simulink model "SLUGS2"  (R2015a)
settings: Solver=FixedStepDiscrete  StartTime=0.0  StopTime=10.0  FixedStep=T  RelTol=1e-3
PreLoadFcn:
  | %T = 0.0025;
  | MavlinkBus;
  | mcuInit;
  | % Baro Altitude Computation
  | % =========================
  | %basePressure = 98192.64;
  | %baseTemp = 288.215;
  | %lapseRate = -0.00198122;
  | %baseHeight = 0;
values from neighbouring files (symbols this model uses):
  apSampleTime = 0.01    [mcuInit.m]
  latlong_WP = 1    [mcuInit.m]
  mavlink_attitude_t = Simulink.Bus    [MavlinkBusMarcello.m]
  mavlink_gps_raw_int_t = Simulink.Bus    [MavlinkBus.m]    (also in MavlinkBusMarcello.m)
  mavlink_raw_imu_t = Simulink.Bus    [MavlinkBus.m]    (also in MavlinkBusMarcello.m)
  mavlink_scaled_pressure_t = Simulink.Bus    [MavlinkBus.m]    (also in MavlinkBusMarcello.m)
  mavlink_servo_output_raw_t = Simulink.Bus    [MavlinkBusMarcello.m]
  mavlink_slugs_navigation_t = Simulink.Bus    [MavlinkBusMarcello.m]
  mavlink_sys_status_t = Simulink.Bus    [MavlinkBus.m]    (also in MavlinkBusMarcello.m)
  SYS_ID_DEF = mpt.Parameter    [mcuInit.m]
  T = 0.01    [mcuInit.m]
  Xpoints = [0 0]    [mcuInit.m]
  Ypoints = [0 0]    [mcuInit.m]
  Zpoints = [0 0]    [mcuInit.m]
undefined symbols (not defined in the file or in its folder): A0, A14, A15, A2, A3, A4, A5, A6, accBiasRateLimit, B0, bankCommandLimit, barAdjust, baroCutoff, baroCutTemp, baseHeight, baseTemp, bdt, cubeAccelGain16405, cubeGyroGain16405, cubeMagGain16405, D0, D11, D7, D8, daLimit, data, daTrimMax, daTrimMin, deLimit, deTrimMax, deTrimMin, drLimit, drTrimMax, drTrimMin, dtLimit, dtTrimMax, dtTrimMin, F2, F3, G0, G13, G15, gaind, GS_location, gyroBiasRateLimit, imuOffset_xacc, imuOffset_xgyro, imuOffset_yacc, imuOffset_ygyro, imuOffset_zacc, imuOffset_zgyro, IPStar, ISA_g, Max, maxAcc, MaxDwnPthStar, maxDynPressure, maxEta, mdt, mlParamInterface ... (+34)
undefined symbols (not defined in the file): baroOffset, baroScale, barTGain1, barTGain2, barTMean1, barTMean2, bda, bde, bdr, bICda, bICde, bICdr, bICdt, derivativesConstant, lapseRate, lowRateSensorCutoff, mainSensorCutoff, mda, mde, mdr, mICda, mICde, mICdr, mICdt, pitotOffset, pitotScale, pitTGain1, pitTGain2, pitTMean1, pitTMean2, powerOffset, powerScale, pressureSensorCutoff, tempOffset, tempScale, vzCutoff, xCutoff, yCutoff
libraries: MCHP_Blockset x151, simulink x84, SLUGS_Library x31, aerolibconvert2 x6, aerolibutil x4, aerolibtransform2 x3, dspmtrx3 x2, aerolibobsolete x2
(part 19 of 24)

== system SLUGS2/Sensor_Data_Adapter/Sensor Suite/If no HIL then Read all the Sensors/if GPS is Ublox ==
  Enable : EnablePort
  Produce the GPS Main Data and update the AP State (lat lon hei cog sog) [gpsUblox.c]1 : MCHP_Blockset/User Functions/C Function Call  ParseFilesChkbx=on  ListFunctions1=Custom Function  Function1=void getGpsUbloxMainData(real32_T* y1);  AddHeaderDeclaration=on  Function1Type=when block is updated (default)  FctReturnBlockOut=off  Fct1BlockOut=y1[5]  DataCollected="s.chksm=reshape({ '638530-ספט-2016 08:52:24','251930-ספט-2016 08:52:57','1628430-ספט-2016 08:52:57','3862408-אוק-2016 23:39:15','360330-ספט-2016 08:52:57','7293730-ספט-2016 08:52:57','954930-ספט-2016 08:52:57','296108-אוק-2016 23:39:15','278130-ספט-2016 08:52:57','556030-ספט-2016 08:52:57','963230-ספט-2016 08:52:57','1122730-ספט-2016 08:52:57','372430-ספט-2016 08:52:57','998830-ספט-2016 08:52:57','522508-אוק-2016 23:39:15'},1,15);s.File1=reshape({ '  void  newCircBuffer(CBRef cB)','  void  freeCircBuffer(CBRef* cB)','  void  freeCircBuffer(CBRef* cB)',' unsigned int  getLength(CBRef cB)','  int  readHead(CBRef cB)','  int  readTail(CBRef cB)',' unsigned char  peak(CBRef cB)',' unsigned char  readFront(CBRef cB)',' unsigned char  writeBack(CBRef cB, unsigned char data)','  void  makeEmpty(CBRef cB)','  void  printCircBuf(CBRef cB)'},1,11);s.File2=reshape({ '  void  uartBufferInit(void)','  void  __attribute__((__interrupt__, no_auto_psv)) _U4RXInterrupt(void)','  void  getGPSRawData(unsigned char* gpsBuffer)',' unsigned char  isGPSNovatel(void)'},1,4);s.File3=reshape({ '  char  hex2char(char halfhex)','  float  degMinToDeg(unsigned char degrees, float minutes)',' unsigned char  gpsUbloxSeparate(unsigned char* outStream)','  void  gpsUbloxParse(void)','  void  getGpsUbloxMainData(float* data)','  char  gpSmbl(char symbl)',' unsigned char  myTokenizer(char* stringToTokenize, char token, char * returnToken)','  void  parseRMC(unsigned char* stream)','  void  parseGGA(unsigned char* stream)',' unsigned char  getChecksum(unsigned char* sentence, unsigned char size)','  void  gpsDebugMsg(unsigned char buf)'},1,11);s.File4=reshape({ '  void  uartMavlinkBufferInit(void)','  void __attribute__((__interrupt__,__auto_psv__)) _U1RXInterrupt(void)','  uint8_t  isFinite(float s)','  void  InitParameterInterface(void)','  void  protDecodeMavlink(void)','  uint16_t  MissionInterfaceResponse(uint8_t system_id, uint8_t component_id)','  uint16_t  ParameterInterfaceResponse(uint8_t system_id, uint8_t component_id)','  uint16_t  PackHeartBeat(uint8_t system_id, uint8_t component_id)','  uint16_t  PackTextMsg(uint8_t system_id, uint8_t component_id, unsigned char buf)','  uint16_t  PackRawIMU(uint8_t system_id, uint8_t component_id, mavlink_raw_imu_t mlRawIMUData ,uint32_t time_usec)','  uint16_t  PackRawAttitude(uint8_t system_id, uint8_t component_id, mavlink_attitude_t mlAttitudeData ,uint32_t time_usec)','  uint16_t  PackGpsRawInt(uint8_t system_id, uint8_t component_id, mavlink_gps_raw_int_t mlRawGpsDataInt ,uint32_t time_usec)','  uint16_t  PackScaledPressure(uint8_t system_id, uint8_t component_id, mavlink_scaled_pressure_t mlAirData ,uint32_t time_usec)','  uint16_t  PackSysStatus(uint8_t system_id, uint8_t component_id, mavlink_sys_status_t mlSysStatus)','  uint16_t  PackRawServo(uint8_t system_id, uint8_t component_id, mavlink_servo_output_raw_t mlPwmCommands ,uint32_t time_usec)','  uint16_t  HIL_PackRawServo(uint8_t system_id, uint8_t component_id, mavlink_servo_output_raw_t mlPwmCommands ,uint32_t time_usec)','  uint16_t  PackRawRC(uint8_t system_id, uint8_t component_id, mavlink_rc_channels_raw_t mlRC_Commands ,uint32_t time_usec)','  uint16_t  PackVFR_HUD(uint8_t system_id, uint8_t component_id, mavlink_vfr_hud_t mlVfr_hud ,uint32_t time_usec)','  char  sendQGCDebugMessage(const char * dbgMessage, char severity, unsigned char* bytesToAdd, char positionStart)','  void  TxN_Data_OverU1(uint16_t N)','  void  TxN_Data_OverU4(uint16_t N)'},1,21);s.File5=reshape({ '  float  myAtan2(float num, float denom)','  float  myPow(float x, float toTheN)','  float  mySqrt(float x)','  float  myAbs(float x)','  float  myAtan(float x)','  float  myAsin(float x)','  float  mySin(float x)','  float  myCos(float x)','  float  myTan(float x)','  float  myAcos(float x)','  float  myExp(float x)','  void  hugeDelay(void)','  void  smallDelay(void)','  void  tinyDelay(void)','  void  printToUart2(const char *fmt, ...)'},1,15);s.File6=reshape({ '  void  sendTelemetryMavlink(unsigned char* dataOut)','  void  uart2Init(void)','  void  gsRead(unsigned char* gsChunk)','  void  prepareTelemetryMavlink(unsigned char* dataOut)','  void  prepareTelemetryMavlink(unsigned char* dataOut)','  void  sendTelemetryMavlink(unsigned char* dataOut)','  void  copyBufferToDMA1(unsigned char size)','  void  send2GS(unsigned char* protData)','  uint8_t  clearWaypointsFrom(uint8_t startingWp)','  void  addMessageToSpiOut(mavlink_message_t* msg)'},1,10);s.File7={ '  void  populateParameterInterface(void)'};s.File8={ '  void  mavlinkInit(void)'};s.File9=reshape({ '  void  updatePWM(unsigned short * PWMData)','  void  updatePWMTrim(unsigned short PWMData, unsigned char channel)','  void  updateLoad(uint8_t mcuLoad)','  void  updateEuler(float* newEuler)','  void  updatePQR(float* newPQR)',' unsigned char  getHilOnOff(void)','  uint8_t  getLightsOnOff(void)','  uint8_t  getLightsDayNight(void)','  void  updateVISensor(uint16_t* data)','  void  updatePTZ(int16_t* ptz)'},1,10);s.File10=reshape({ '  void  updateRawADCData(int16_t* adcData)','  void  updateAirData(float* airData)','  void  updateLoadData(uint8_t load, uint16_t mvPower)','  void  updateAttitude(float * attitudeData)','  void  getGSLocation(float* altLatLon)','  void  updateTimeStamp(uint32_t timeSt)','  void  updatePosition(float * posData)','  void  updatePilotConsole(uint16_t * pilData)','  void  updateDiagnosticFl(float* diagFl)','  void  updateDiagnosticSh(int16_t* diagSh)','  void  updateBias(float * biasData)','  void  updateSensorData(float* sens)','  uint8_t  isFixValid(void)','  void  updateSensorDiag(float* diag)'},1,14);s.File11=reshape({ '  void  gpsInit(void)','  void  gpsParse(uint8_t* dataStream)','  void  updateStatus(uint8_t* completeMessage)','  void  updatePositionData(uint8_t* completeMessage)','  void  updateVelocityData(uint8_t* completeMessage)','  void  updateTimeData(uint8_t* completeMessage)','  void  getGpsMainData(float* data)','  uint32_t  CRC32Value(int32_t i)','  uint32_t  CalculateBlockCRC32(uint32_t ulCount, uint8_t *ucBuffer)','  uint16_t  charsToUint16(uint8_t* data)','  uint32_t  charsToUint32(uint8_t* data)','  float  charsToFloat(uint8_t* data)','  double  charsToDouble(uint8_t* data)'},1,13);s.File12=reshape({ '  void  getMidLevelCommands(float* commands)',' unsigned char  isApManual(uint16_t failsafe)','  float  getParamIdx(unsigned char idx)','  void  getRangeOfParams(uint8_t startIdx, uint8_t endIdx, float* parameters)','  float  getDynamic(void)','  void  getAttitude(float* attitude)','  void  getXYZ(float* xyz)','  void  getVned(float* xyz)','  uint8_t  getMaxWp(void)',' unsigned char  isWpFly(void)',' unsigned char  isPassthrough(void)','  void  setDiagnosticFloat(float * flValues)','  void  setDiagnosticShort(int16_t* shValues)','  void  getWP(unsigned char idx, float* WPpos)','  void  setLogFloat1(float * flValues)','  void  setLogFloat2(float * flValues)',' unsigned char  getApControlType(void)',' unsigned char  getPassValues(uint8_t* pasVals)','  void  setCurrentCommands(float airSpeed)','  void  getCurrentGPSPos(float* latLonAlt)','  void  setNavLong(float* values)','  void  setNavLat(float* values)','  void  setNavNav(float* values)','  void  getAccels(float * accels)','  void  getAccBias(float * bias)','  void  getRTB(uint8_t* rtb)','  void  getMobileLocation(float* loc)','  uint8_t  getNavMode(void)','  void  getISRLocation(float* loc)','  uint8_t  getISRCameraOption1(void)',' unsigned short  meanFilter5(unsigned short * values)','  uint8_t  justEnabled(uint8_t enableValue, uint8_t index)',' unsigned char  quickSort(unsigned short *arr, char elements)'},1,33);s.File13=reshape({ '  void  hilRead(unsigned char* hilChunk)','  void  hil_getRawRead(short * rawData)','  void  hil_getVned(float* vned)','  void  hil_getEuler(float* euler)','  void  hil_getRates(float* pqr)','  void  hil_getXYZ(float* xyz)',' unsigned int  hil_getTs(void)','  void  protDecodeHil(uint8_t* dataIn)'},1,8);s.File14=reshape({ '  void  cubeInit(void)','  void  getCubeData(short * cubeData)','  void  updateCubeData(void)','  int16_t  averageData(int16_t* theData, uint8_t count)',' unsigned short  write2Cube(unsigned short data2Send)','  short  convert14BitToShort(short wordData)','  short  convert12BitToShort(short wordData)',' unsigned char  isCube16405(void)'},1,8);s.File15=reshape({ '  void  uartMavlinkBufferInit(void)','  uint16_t  PackHeartBeat(uint8_t system_id, uint8_t component_id)','  uint16_t  PackRawServo(uint8_t system_id, uint8_t component_id, mavlink_servo_output_raw_t mlPwmCommands ,uint32_t time_usec)','  uint16_t  HIL_PackRawServo(uint8_t system_id, uint8_t component_id, mavlink_servo_output_raw_t mlPwmCommands ,uint32_t time_usec)','  uint16_t  PackRawRC(uint8_t system_id, uint8_t component_id, mavlink_rc_channels_raw_t mlRC_Commands, uint32_t time_usec)','  uint16_t  PackVFR_HUD(uint8_t system_id, uint8_t component_id, mavlink_vfr_hud_t mlVfr_hud, uint32_t time_usec)','  uint16_t  PackRawIMU(uint8_t system_id, uint8_t component_id, mavlink_raw_imu_t mlRawIMUData ,uint32_t time_usec)','  uint16_t  PackRawAttitude(uint8_t system_id, uint8_t component_id, mavlink_attitude_t mlAttitudeData ,uint32_t time_usec)','  char  sendQGCDebugMessage(const char * dbgMessage, char severity, unsigned char* bytesToAdd, char positionStart)','  uint16_t  PackGpsRawInt(uint8_t system_id, uint8_t component_id, mavlink_gps_raw_int_t mlRawGpsDataInt, uint32_t time_usec)','  uint16_t  PackScaledPressure(uint8_t system_id, uint8_t component_id, mavlink_scaled_pressure_t mlAirData, uint32_t time_usec)','  uint16_t  PackSysStatus(uint8_t system_id, uint8_t component_id, mavlink_sys_status_t mlSysStatus)'},1,12);"  ORDERING=None  SampleTime=.01  MCHP_MASTERLINK=|  PinDigitalInput=[]  PinDigitalOutput=[]  PinAnalogInput=[]
      | SLUGS2/Microchip Master
      | AUAV V3 Board
      | Busy Flag on D2 (RA6)
  GPS Main : Outport
  wires:
  Produce the GPS Main Data and update the AP State (lat lon hei cog sog) [gpsUblox.c]1/1 -> GPS Main/1

== system SLUGS2/Sensor_Data_Adapter/Sensor Suite/Low Pass Filtering,Temperature Compensation and Calibration/Baro Altimeter ==
  Static (Pa) : Inport
  Compute Barometric Height : Subsystem  mask{baseTemp=baseTemp, LapseRate=lapseRate}
      mask prompts: baseTemp "Base Station Temperature (K)"; LapseRate "Lapse Rate (C/ft)"
      mask help:
      | Produces Altitude in meters from Barometric Pressure in Pascals. Altitude is valid from MSL to 6000 ft.
      |
      | The method implemented here was developed by Ren Curry
  Enabled Subsystem : Subsystem  TreatAsAtomicUnit=on
  Enables/Disables the Computation of initial Baro Bias : MATLAB Function  TreatAsAtomicUnit=on
  GS Height : Subsystem
  Initial Baro Bias : Subsystem  TreatAsAtomicUnit=on
  Logical Operator : Logic  Operator=NOT  AllPortsSameDT=off  OutDataTypeStr=boolean
  Sum1 : Sum  Inputs=++|  OutDataTypeStr=single
  Zero Out Height : Subsystem  TreatAsAtomicUnit=on
  Altitude : Outport
  wires:
  Compute Barometric Height/1("Altitude, m") -> Zero Out Height/2(Computed Height), Sum1/2
  Static (Pa)/1 -> Initial Baro Bias/1(Baro (Pa)), Compute Barometric Height/3(Baro (Pa))
  Enables/Disables the Computation of initial Baro Bias/1(tOut) -> Initial Baro Bias/Enable, Zero Out Height/Enable, Logical Operator/1
  GS Height/1(GS Height) -> Compute Barometric Height/1(Base Height (m)), Zero Out Height/1(Base Height)
  Initial Baro Bias/1(Baro (Gnd)) -> Compute Barometric Height/2(Base Pressure (Pa))
  Zero Out Height/1(Height Offset) -> Sum1/1
  Logical Operator/1 -> Enabled Subsystem/Enable
  Sum1/1 -> Enabled Subsystem/1(In1)
  Enabled Subsystem/1(Out1) -> Altitude/1

== system SLUGS2/Sensor_Data_Adapter/Sensor Suite/Low Pass Filtering,Temperature Compensation and Calibration/Barometer Unit Conversion ==
  Raw : Inport
  Bias : Constant  Value=bias  OutDataTypeStr=single
  Divide : Product  OutDataTypeStr=single
  Gains : Constant  Value=gains  OutDataTypeStr=single
  Sum : Sum  Inputs=|++  OutDataTypeStr=single
  Comp : Outport
  wires:
  Bias/1 -> Sum/2
  Raw/1 -> Divide/2
  Gains/1 -> Divide/1
  Divide/1 -> Sum/1
  Sum/1 -> Comp/1

== system SLUGS2/Sensor_Data_Adapter/Sensor Suite/Low Pass Filtering,Temperature Compensation and Calibration/Pitot Unit Conversion ==
  Raw : Inport
  Bias : Constant  Value=bias  OutDataTypeStr=single
  Divide : Product  OutDataTypeStr=single
  Gains : Constant  Value=gains  OutDataTypeStr=single
  Sum : Sum  Inputs=|++  OutDataTypeStr=single
  Comp : Outport
  wires:
  Bias/1 -> Sum/2
  Raw/1 -> Divide/2
  Gains/1 -> Divide/1
  Divide/1 -> Sum/1
  Sum/1 -> Comp/1

== system SLUGS2/Sensor_Data_Adapter/Sensor Suite/Low Pass Filtering,Temperature Compensation and Calibration/Power Unit Conversion ==
  Raw : Inport
  Bias : Constant  Value=bias  OutDataTypeStr=single
  Divide : Product  OutDataTypeStr=single
  Gains : Constant  Value=gains  OutDataTypeStr=single
  Sum : Sum  Inputs=|++  OutDataTypeStr=single
  Comp : Outport
  wires:
  Bias/1 -> Sum/2
  Raw/1 -> Divide/2
  Gains/1 -> Divide/1
  Divide/1 -> Sum/1
  Sum/1 -> Comp/1

== system SLUGS2/Sensor_Data_Adapter/Sensor Suite/Low Pass Filtering,Temperature Compensation and Calibration/Temp Compensate Accel X1 ==
  Temp : Inport
  Dynamic : Inport  Port=2
  Compare To Constant : simulink/Logic and Bit Operations/Compare To Constant  relop=<  const=pitCutTemp  OutDataTypeStr=uint8  ZeroCross=off
  Display : Display
  Display2 : Display
  Hi Temp Compensation2 : Subsystem  mask{alpha=pitTGain2, tempMean=pitTMean2}
      mask prompts: alpha "Tempearature Coeficient (K_t)"; tempMean "Calibration Temperature Mean (T_avg)"
      mask help:
      | This block implements a temperature compensation. It implmements the following equation:
      |
      | M_tc = M_raw - K_t(T - T_avg)
  Lo Temp Compensation : Subsystem  mask{alpha=pitTGain1, tempMean=pitTMean1}
      mask prompts: alpha "Tempearature Coeficient (K_t)"; tempMean "Calibration Temperature Mean (T_avg)"
      mask help:
      | This block implements a temperature compensation. It implmements the following equation:
      |
      | M_tc = M_raw - K_t(T - T_avg)
  Logical Operator : Logic  Operator=NOT  AllPortsSameDT=off  OutDataTypeStr=boolean
  Merge : Merge
  Baro_c : Outport
  wires:
  Hi Temp Compensation2/1(Comp) -> Merge/1
  Logical Operator/1 -> Hi Temp Compensation2/Enable, Display2/1
  Merge/1 -> Baro_c/1, Display/1
  Dynamic/1 -> Lo Temp Compensation/1(Raw), Hi Temp Compensation2/1(Raw)
  Temp/1 -> Compare To Constant/1, Lo Temp Compensation/2(Temp Raw), Hi Temp Compensation2/2(Temp Raw)
  Compare To Constant/1 -> Lo Temp Compensation/Enable, Logical Operator/1
  Lo Temp Compensation/1(Comp) -> Merge/2

== system SLUGS2/Sensor_Data_Adapter/Sensor Suite/Low Pass Filtering,Temperature Compensation and Calibration/Temp Compensate Baro ==
  Temp : Inport
  Baro : Inport  Port=2
  Compare To Constant : simulink/Logic and Bit Operations/Compare To Constant  relop=<  const=baroCutTemp  OutDataTypeStr=uint8  ZeroCross=off
  Hi Temp Compensation : Subsystem  mask{alpha=barTGain2, tempMean=barTMean2}
      mask prompts: alpha "Tempearature Coeficient (K_t)"; tempMean "Calibration Temperature Mean (T_avg)"
      mask help:
      | This block implements a temperature compensation. It implmements the following equation:
      |
      | M_tc = M_raw - K_t(T - T_avg)
  Lo Temp Compensation : Subsystem  mask{alpha=barTGain1, tempMean=barTMean1}
      mask prompts: alpha "Tempearature Coeficient (K_t)"; tempMean "Calibration Temperature Mean (T_avg)"
      mask help:
      | This block implements a temperature compensation. It implmements the following equation:
      |
      | M_tc = M_raw - K_t(T - T_avg)
  Logical Operator : Logic  Operator=NOT  AllPortsSameDT=off  OutDataTypeStr=boolean
  Merge : Merge
  Baro_c : Outport
  wires:
  Compare To Constant/1 -> Logical Operator/1, Lo Temp Compensation/Enable
  Temp/1 -> Compare To Constant/1, Hi Temp Compensation/2(Temp Raw), Lo Temp Compensation/2(Temp Raw)
  Baro/1 -> Hi Temp Compensation/1(Raw), Lo Temp Compensation/1(Raw)
  Lo Temp Compensation/1(Comp) -> Merge/2
  Merge/1 -> Baro_c/1
  Logical Operator/1 -> Hi Temp Compensation/Enable
  Hi Temp Compensation/1(Comp) -> Merge/1

== system SLUGS2/Sensor_Data_Adapter/Sensor Suite/Low Pass Filtering,Temperature Compensation and Calibration/Thermistor Unit Conversion ==
  Raw : Inport
  Bias : Constant  Value=bias  OutDataTypeStr=single
  Divide : Product  OutDataTypeStr=single
  Gains : Constant  Value=gains  OutDataTypeStr=single
  Sum : Sum  Inputs=|++  OutDataTypeStr=single
  Comp : Outport
  wires:
  Sum/1 -> Comp/1
  Divide/1 -> Sum/1
  Gains/1 -> Divide/1
  Raw/1 -> Divide/2
  Bias/1 -> Sum/2

== system SLUGS2/Sensor_Data_Adapter/Sensor Suite/Low Pass Filtering,Temperature Compensation and Calibration/Tustin Lowpass, Auto Initial Condition1 ==
  In1 : Inport
  Constant : Constant  Value=T
  Constant1 : Constant  Value=f
  Embedded MATLAB Function : MATLAB Function  TreatAsAtomicUnit=on
  Out1 : Outport
  wires:
  Constant/1 -> Embedded MATLAB Function/2(T)
  Constant1/1 -> Embedded MATLAB Function/3(f)
  Embedded MATLAB Function/1(y) -> Out1/1
  In1/1 -> Embedded MATLAB Function/1(u)

== system SLUGS2/Sensor_Data_Adapter/Sensor Suite/Low Pass Filtering,Temperature Compensation and Calibration/Tustin Lowpass, Auto Initial Condition2 ==
  In1 : Inport
  Constant : Constant  Value=T
  Constant1 : Constant  Value=f
  Embedded MATLAB Function : MATLAB Function  TreatAsAtomicUnit=on
  Out1 : Outport
  wires:
  In1/1 -> Embedded MATLAB Function/1(u)
  Embedded MATLAB Function/1(y) -> Out1/1
  Constant1/1 -> Embedded MATLAB Function/3(f)
  Constant/1 -> Embedded MATLAB Function/2(T)

== system SLUGS2/Sensor_Data_Adapter/Sensor Suite/Low Pass Filtering,Temperature Compensation and Calibration/Tustin Lowpass, Auto Initial Condition3 ==
  In1 : Inport
  Constant : Constant  Value=T
  Constant1 : Constant  Value=f
  Embedded MATLAB Function : MATLAB Function  TreatAsAtomicUnit=on
  Out1 : Outport
  wires:
  Constant/1 -> Embedded MATLAB Function/2(T)
  Constant1/1 -> Embedded MATLAB Function/3(f)
  Embedded MATLAB Function/1(y) -> Out1/1
  In1/1 -> Embedded MATLAB Function/1(u)

== system SLUGS2/Sensor_Data_Adapter/Sensor Suite/Low Pass Filtering,Temperature Compensation and Calibration/Tustin Lowpass, Auto Initial Condition4 ==
  In1 : Inport
  Constant : Constant  Value=T
  Constant1 : Constant  Value=f
  Embedded MATLAB Function : MATLAB Function  TreatAsAtomicUnit=on
  Out1 : Outport
  wires:
  In1/1 -> Embedded MATLAB Function/1(u)
  Embedded MATLAB Function/1(y) -> Out1/1
  Constant1/1 -> Embedded MATLAB Function/3(f)
  Constant/1 -> Embedded MATLAB Function/2(T)

== system SLUGS2/Update PWM Commands and Send Telemetry [updated 4.27.16]/Generate PWM Signals Based on the Control Type/If  Control Type Is Selective Passthrough/Convert to PWM ==
  " Angle(rad)" : Inport
  Add : Sum
  Constant1 : Constant  Value=slopem
  Constant2 : Constant  Value=interceptb
  Data Type Conversion : DataTypeConversion  OutDataTypeStr=uint16
  Divide : Product
  PWM : Outport
  wires:
  Data Type Conversion/1 -> PWM/1
  " Angle(rad)"/1 -> Divide/1
  Constant2/1 -> Add/2
  Divide/1 -> Add/1
  Add/1 -> Data Type Conversion/1
  Constant1/1 -> Divide/2

== system SLUGS2/Update PWM Commands and Send Telemetry [updated 4.27.16]/Generate PWM Signals Based on the Control Type/If  Control Type Is Selective Passthrough/Convert to PWM1 ==
  " Angle(rad)" : Inport
  Add : Sum
  Constant1 : Constant  Value=slopem
  Constant2 : Constant  Value=interceptb
  Data Type Conversion : DataTypeConversion  OutDataTypeStr=uint16
  Divide : Product
  PWM : Outport
  wires:
  Constant1/1 -> Divide/2
  Add/1 -> Data Type Conversion/1
  Divide/1 -> Add/1
  Constant2/1 -> Add/2
  " Angle(rad)"/1 -> Divide/1
  Data Type Conversion/1 -> PWM/1

== system SLUGS2/Update PWM Commands and Send Telemetry [updated 4.27.16]/Generate PWM Signals Based on the Control Type/If  Control Type Is Selective Passthrough/Convert to PWM2 ==
  " Angle(rad)" : Inport
  Add : Sum
  Constant1 : Constant  Value=slopem
  Constant2 : Constant  Value=interceptb
  Data Type Conversion : DataTypeConversion  OutDataTypeStr=uint16
  Divide : Product
  PWM : Outport
  wires:
  Data Type Conversion/1 -> PWM/1
  " Angle(rad)"/1 -> Divide/1
  Constant2/1 -> Add/2
  Divide/1 -> Add/1
  Add/1 -> Data Type Conversion/1
  Constant1/1 -> Divide/2

== system SLUGS2/Update PWM Commands and Send Telemetry [updated 4.27.16]/Generate PWM Signals Based on the Control Type/If  Control Type Is Selective Passthrough/Convert to PWM3 ==
  " Angle(rad)" : Inport
  Add : Sum
  Constant1 : Constant  Value=slopem
  Constant2 : Constant  Value=interceptb
  Data Type Conversion : DataTypeConversion  OutDataTypeStr=uint16
  Divide : Product
  PWM : Outport
  wires:
  Constant1/1 -> Divide/2
  Add/1 -> Data Type Conversion/1
  Divide/1 -> Add/1
  Constant2/1 -> Add/2
  " Angle(rad)"/1 -> Divide/1
  Data Type Conversion/1 -> PWM/1

== system SLUGS2/Update PWM Commands and Send Telemetry [updated 4.27.16]/Generate PWM Signals Based on the Control Type/If  Control Type Is Wp, ISR, LP or  Mid Lvl Cmds/Convert to PWM ==
  " Angle(rad)" : Inport
  Add : Sum
  Constant1 : Constant  Value=slopem
  Constant2 : Constant  Value=interceptb
  Data Type Conversion : DataTypeConversion  OutDataTypeStr=uint16
  Divide : Product
  PWM : Outport
  wires:
  Data Type Conversion/1 -> PWM/1
  " Angle(rad)"/1 -> Divide/1
  Constant2/1 -> Add/2
  Divide/1 -> Add/1
  Add/1 -> Data Type Conversion/1
  Constant1/1 -> Divide/2

== system SLUGS2/Update PWM Commands and Send Telemetry [updated 4.27.16]/Generate PWM Signals Based on the Control Type/If  Control Type Is Wp, ISR, LP or  Mid Lvl Cmds/Convert to PWM1 ==
  " Angle(rad)" : Inport
  Add : Sum
  Constant1 : Constant  Value=slopem
  Constant2 : Constant  Value=interceptb
  Data Type Conversion : DataTypeConversion  OutDataTypeStr=uint16
  Divide : Product
  PWM : Outport
  wires:
  Constant1/1 -> Divide/2
  Add/1 -> Data Type Conversion/1
  Divide/1 -> Add/1
  Constant2/1 -> Add/2
  " Angle(rad)"/1 -> Divide/1
  Data Type Conversion/1 -> PWM/1

== system SLUGS2/Update PWM Commands and Send Telemetry [updated 4.27.16]/Generate PWM Signals Based on the Control Type/If  Control Type Is Wp, ISR, LP or  Mid Lvl Cmds/Convert to PWM2 ==
  " Angle(rad)" : Inport
  Add : Sum
  Constant1 : Constant  Value=slopem
  Constant2 : Constant  Value=interceptb
  Data Type Conversion : DataTypeConversion  OutDataTypeStr=uint16
  Divide : Product
  PWM : Outport
  wires:
  Data Type Conversion/1 -> PWM/1
  " Angle(rad)"/1 -> Divide/1
  Constant2/1 -> Add/2
  Divide/1 -> Add/1
  Add/1 -> Data Type Conversion/1
  Constant1/1 -> Divide/2

== system SLUGS2/Update PWM Commands and Send Telemetry [updated 4.27.16]/Generate PWM Signals Based on the Control Type/If  Control Type Is Wp, ISR, LP or  Mid Lvl Cmds/Convert to PWM3 ==
  " Angle(rad)" : Inport
  Add : Sum
  Constant1 : Constant  Value=slopem
  Constant2 : Constant  Value=interceptb
  Data Type Conversion : DataTypeConversion  OutDataTypeStr=uint16
  Divide : Product
  PWM : Outport
  wires:
  Constant1/1 -> Divide/2
  Add/1 -> Data Type Conversion/1
  Divide/1 -> Add/1
  Constant2/1 -> Add/2
  " Angle(rad)"/1 -> Divide/1
  Data Type Conversion/1 -> PWM/1

== system SLUGS2/Update PWM Commands and Send Telemetry [updated 4.27.16]/Generate PWM Signals Based on the Control Type/If  Control Type Is Wp, ISR, LP or  Mid Lvl Cmds and we want to add Selective Passthrough1/Average ==
  In1 : Inport
  In2 : Inport  Port=2
  Add : Sum
  Gain4 : Gain  Gain=1/2
  Out1 : Outport
  wires:
  In1/1 -> Add/1
  Gain4/1 -> Out1/1
  Add/1 -> Gain4/1
  In2/1 -> Add/2

== system SLUGS2/Update PWM Commands and Send Telemetry [updated 4.27.16]/Generate PWM Signals Based on the Control Type/If  Control Type Is Wp, ISR, LP or  Mid Lvl Cmds and we want to add Selective Passthrough1/Average1 ==
  In1 : Inport
  In2 : Inport  Port=2
  Add : Sum
  Gain4 : Gain  Gain=1/2
  Out1 : Outport
  wires:
  In1/1 -> Add/1
  Gain4/1 -> Out1/1
  Add/1 -> Gain4/1
  In2/1 -> Add/2

== system SLUGS2/Update PWM Commands and Send Telemetry [updated 4.27.16]/Generate PWM Signals Based on the Control Type/If  Control Type Is Wp, ISR, LP or  Mid Lvl Cmds and we want to add Selective Passthrough1/Average2 ==
  In1 : Inport
  In2 : Inport  Port=2
  Add : Sum
  Gain4 : Gain  Gain=1/2
  Out1 : Outport
  wires:
  In1/1 -> Add/1
  Gain4/1 -> Out1/1
  Add/1 -> Gain4/1
  In2/1 -> Add/2

== system SLUGS2/Update PWM Commands and Send Telemetry [updated 4.27.16]/Generate PWM Signals Based on the Control Type/If  Control Type Is Wp, ISR, LP or  Mid Lvl Cmds and we want to add Selective Passthrough1/Average3 ==
  In1 : Inport
  In2 : Inport  Port=2
  Add : Sum
  Gain4 : Gain  Gain=1/2
  Out1 : Outport
  wires:
  In1/1 -> Add/1
  Gain4/1 -> Out1/1
  Add/1 -> Gain4/1
  In2/1 -> Add/2

== system SLUGS2/Update PWM Commands and Send Telemetry [updated 4.27.16]/Generate PWM Signals Based on the Control Type/If  Control Type Is Wp, ISR, LP or  Mid Lvl Cmds and we want to add Selective Passthrough1/Convert to PWM ==
  " Angle(rad)" : Inport
  Add : Sum
  Constant1 : Constant  Value=slopem
  Constant2 : Constant  Value=interceptb
  Data Type Conversion : DataTypeConversion  OutDataTypeStr=uint16
  Divide : Product
  PWM : Outport
  wires:
  Data Type Conversion/1 -> PWM/1
  " Angle(rad)"/1 -> Divide/1
  Constant2/1 -> Add/2
  Divide/1 -> Add/1
  Add/1 -> Data Type Conversion/1
  Constant1/1 -> Divide/2

== system SLUGS2/Update PWM Commands and Send Telemetry [updated 4.27.16]/Generate PWM Signals Based on the Control Type/If  Control Type Is Wp, ISR, LP or  Mid Lvl Cmds and we want to add Selective Passthrough1/Convert to PWM1 ==
  " Angle(rad)" : Inport
  Add : Sum
  Constant1 : Constant  Value=slopem
  Constant2 : Constant  Value=interceptb
  Data Type Conversion : DataTypeConversion  OutDataTypeStr=uint16
  Divide : Product
  PWM : Outport
  wires:
  Constant1/1 -> Divide/2
  Add/1 -> Data Type Conversion/1
  Divide/1 -> Add/1
  Constant2/1 -> Add/2
  " Angle(rad)"/1 -> Divide/1
  Data Type Conversion/1 -> PWM/1

== system SLUGS2/Update PWM Commands and Send Telemetry [updated 4.27.16]/Generate PWM Signals Based on the Control Type/If  Control Type Is Wp, ISR, LP or  Mid Lvl Cmds and we want to add Selective Passthrough1/Convert to PWM2 ==
  " Angle(rad)" : Inport
  Add : Sum
  Constant1 : Constant  Value=slopem
  Constant2 : Constant  Value=interceptb
  Data Type Conversion : DataTypeConversion  OutDataTypeStr=uint16
  Divide : Product
  PWM : Outport
  wires:
  Data Type Conversion/1 -> PWM/1
  " Angle(rad)"/1 -> Divide/1
  Constant2/1 -> Add/2
  Divide/1 -> Add/1
  Add/1 -> Data Type Conversion/1
  Constant1/1 -> Divide/2

== system SLUGS2/Update PWM Commands and Send Telemetry [updated 4.27.16]/Generate PWM Signals Based on the Control Type/If  Control Type Is Wp, ISR, LP or  Mid Lvl Cmds and we want to add Selective Passthrough1/Convert to PWM3 ==
  " Angle(rad)" : Inport
  Add : Sum
  Constant1 : Constant  Value=slopem
  Constant2 : Constant  Value=interceptb
  Data Type Conversion : DataTypeConversion  OutDataTypeStr=uint16
  Divide : Product
  PWM : Outport
  wires:
  Constant1/1 -> Divide/2
  Add/1 -> Data Type Conversion/1
  Divide/1 -> Add/1
  Constant2/1 -> Add/2
  " Angle(rad)"/1 -> Divide/1
  Data Type Conversion/1 -> PWM/1

== system SLUGS2/Inner Loop// Navigation/L1 Output Feedback Controller With Projection Operator/Control Law/Compute Coef/dsPIC_exp ==
  u : Inport
  Environment Controller : simulink/Signal Routing/Environment Controller
  Math Function : Math  SaturateOnIntegerOverflow=on
  myExp() apUtils.c [updated 5.1.16] : MCHP_Blockset/User Functions/C Function Call  ParseFilesChkbx=off  ListFunctions1=Custom Function  Function1=float myExp(float x)  AddHeaderDeclaration=on  Function1Type=when block is updated (default)  Fct1BlockIn=x  FctReturnBlockOut=on  DataCollected=0  ORDERING=None  SampleTime=-1  MCHP_MASTERLINK=|  PinDigitalInput=[]  PinDigitalOutput=[]  PinAnalogInput=[]
      | SLUGS2/Microchip Master
      | AUAV V3 Board
      | Busy Flag on D2 (RA6)
  exp(u) : Outport
  wires:
  Math Function/1 -> Environment Controller/1
  u/1 -> Math Function/1, myExp() apUtils.c [updated 5.1.16]/1
  Environment Controller/1 -> exp(u)/1
  myExp() apUtils.c [updated 5.1.16]/1 -> Environment Controller/2

== system SLUGS2/Inner Loop// Navigation/L1 Output Feedback Controller With Projection Operator/State Predictor/Compute Coef/dsPIC_exp ==
  u : Inport
  Environment Controller : simulink/Signal Routing/Environment Controller
  Math Function : Math  SaturateOnIntegerOverflow=on
  myExp() apUtils.c [updated 5.1.16] : MCHP_Blockset/User Functions/C Function Call  ParseFilesChkbx=off  ListFunctions1=Custom Function  Function1=float myExp(float x)  AddHeaderDeclaration=on  Function1Type=when block is updated (default)  Fct1BlockIn=x  FctReturnBlockOut=on  DataCollected=0  ORDERING=None  SampleTime=-1  MCHP_MASTERLINK=|  PinDigitalInput=[]  PinDigitalOutput=[]  PinAnalogInput=[]
      | SLUGS2/Microchip Master
      | AUAV V3 Board
      | Busy Flag on D2 (RA6)
  exp(u) : Outport
  wires:
  Math Function/1 -> Environment Controller/1
  u/1 -> Math Function/1, myExp() apUtils.c [updated 5.1.16]/1
  Environment Controller/1 -> exp(u)/1
  myExp() apUtils.c [updated 5.1.16]/1 -> Environment Controller/2

== system SLUGS2/Inner Loop// Navigation/Lateral Channel Encaps [updated 4.28.16]/Lateral Channel/Roll Control [PID]/Trapezoidal Integrator ==
  x : Inport
  Reset : Inport  Port=2
  Constant : Constant  Value=1/3  OutDataTypeStr=single
  Constant1 : Constant  Value=4/3  OutDataTypeStr=single
  Constant2 : Constant  Value=T/2  OutDataTypeStr=single
  Constant3 : Constant  Value=1/3  OutDataTypeStr=single
  Constant5 : Constant  Value=0  OutDataTypeStr=single
  Integer Delay : Delay  DelayLength=1  InputProcessing=Inherited  SampleTime=T
  Integer Delay1 : Delay  InputProcessing=Inherited  SampleTime=T
  Integer Delay2 : Delay  DelayLength=1  InputProcessing=Inherited  SampleTime=T
  Product{,1..3} (4 alike) : Product  OutDataTypeStr=single  RndMeth=Zero
  "Protect NaNs " : Subsystem
  Protect NaNs1 : Subsystem
  Subtract : Sum  Inputs=3  OutDataTypeStr=single
  Subtract1 : Sum  Inputs=2  OutDataTypeStr=single
  Switch1 : Switch  Criteria=u2 > Threshold  Threshold=0.3  SampleTime=.01
  Int(x) : Outport
  wires:
  Switch1/1 -> Protect NaNs1/1(In1)
  Reset/1 -> Switch1/2
  Constant5/1 -> Switch1/1
  Product3/1 -> Subtract1/2
  Integer Delay2/1 -> Subtract1/1
  Subtract1/1 -> Switch1/3
  Subtract/1 -> Product3/2
  Constant2/1 -> Product3/1
  Product2/1 -> Subtract/3
  Product1/1 -> Subtract/2
  Product/1 -> Subtract/1
  x/1 -> "Protect NaNs "/1(In1)
  Constant3/1 -> Product2/2
  Integer Delay1/1 -> Product2/1
  Integer Delay/1 -> Product1/1
  Constant1/1 -> Product1/2
  Constant/1 -> Product/2
  Protect NaNs1/1(Out1) -> Integer Delay2/1, Int(x)/1
  "Protect NaNs "/1(Out1) -> Integer Delay1/1, Integer Delay/1, Product/1

== system SLUGS2/Inner Loop// Navigation/Lateral Channel Encaps [updated 4.28.16]/Lateral Channel/Sideslip Compensation/Bank to Psi Dot ==
  phi_c : Inport
  U_m : Inport  Port=2
  Constant1 : Constant  Value=9.80665  OutDataTypeStr=single
  Divide : Product  Inputs=/*  OutDataTypeStr=single  SampleTime=apSampleTime
  Divide1 : Product  OutDataTypeStr=single  SampleTime=apSampleTime
  bank Limit : Saturate  UpperLimit=bankCommandLimit  LowerLimit=-bankCommandLimit
  dsPIC_tan : Subsystem  AncestorBlock=SLUGS_Library/dsPIC_tan
  negprotect : MATLAB Function  TreatAsAtomicUnit=on
  psi_dot_c : Outport
  wires:
  bank Limit/1 -> dsPIC_tan/1(x)
  negprotect/1(zpVal) -> Divide/1
  Divide/1 -> Divide1/2
  phi_c/1 -> bank Limit/1
  dsPIC_tan/1(tan(x)) -> Divide1/1
  Divide1/1 -> psi_dot_c/1
  Constant1/1 -> Divide/2
  U_m/1 -> negprotect/1(val)

== system SLUGS2/Inner Loop// Navigation/Lateral Channel Encaps [updated 4.28.16]/Lateral Channel/Sideslip Compensation/Low Pass ==
  a : Inport
  u : Inport  Port=2
  Compute Coef : Subsystem
  Detect Change : Subsystem
  Divide : Product  SampleTime=apSampleTime
  Divide1 : Product  SampleTime=apSampleTime
  IC : InitialCondition
  Integer Delay : Delay  DelayLength=1  InputProcessing=Inherited  SampleTime=apSampleTime
  Integer Delay1 : Delay  DelayLength=1  InputProcessing=Inherited  SampleTime=apSampleTime
  Subtract : Sum  SampleTime=apSampleTime
  y : Outport
  wires:
  a/1 -> Compute Coef/1(a), Detect Change/1(Data)
  Compute Coef/1(b) -> Divide/1
  Compute Coef/2(c) -> Divide1/1
  Detect Change/1(change?) -> IC/1
  Integer Delay/1 -> Divide/2
  Divide/1 -> Subtract/1
  Divide1/1 -> Subtract/2
  Subtract/1 -> y/1, Integer Delay1/1
  IC/1 -> Compute Coef/Enable
  u/1 -> Integer Delay/1
  Integer Delay1/1 -> Divide1/2

== system SLUGS2/Inner Loop// Navigation/Lateral Channel Encaps [updated 4.28.16]/Lateral Channel/Sideslip Compensation/Protect NaNs2 ==
  In1 : Inport
  Integer Delay3 : Delay  DelayLength=1  InputProcessing=Inherited  SampleTime=T
  Relational Operator2 : RelationalOperator  Operator===  OutDataTypeStr=uint(8)
  Switch3 : Switch  Criteria=u2 > Threshold  Threshold=0.3  SampleTime=.01
  Out1 : Outport
  wires:
  Integer Delay3/1 -> Switch3/3
  Switch3/1 -> Out1/1, Integer Delay3/1
  In1/1 -> Relational Operator2/2, Relational Operator2/1, Switch3/1
  Relational Operator2/1 -> Switch3/2

== system SLUGS2/Inner Loop// Navigation/Lateral Channel Encaps [updated 4.28.16]/Lateral Channel/Sideslip Compensation/psi_dot to Bank ==
  psi_dot_c : Inport
  U_m : Inport  Port=2
  Constant1 : Constant  Value=9.80665  OutDataTypeStr=single
  Divide : Product  Inputs=**/  SampleTime=apSampleTime
  dsPIC_atan : Subsystem  AncestorBlock=SLUGS_Library/dsPIC_atan
  phi_c : Outport
  wires:
  Divide/1 -> dsPIC_atan/1(x)
  dsPIC_atan/1(atan(x)) -> phi_c/1
  Constant1/1 -> Divide/3
  U_m/1 -> Divide/2
  psi_dot_c/1 -> Divide/1

== system SLUGS2/Inner Loop// Navigation/Lateral Channel Encaps [updated 4.28.16]/Lateral Channel/Yaw Damper [PID]/Trapezoidal Integrator ==
  x : Inport
  Reset : Inport  Port=2
  Constant : Constant  Value=1/3  OutDataTypeStr=single
  Constant1 : Constant  Value=4/3  OutDataTypeStr=single
  Constant2 : Constant  Value=T/2  OutDataTypeStr=single
  Constant3 : Constant  Value=1/3  OutDataTypeStr=single
  Constant5 : Constant  Value=0  OutDataTypeStr=single
  Integer Delay : Delay  DelayLength=1  InputProcessing=Inherited  SampleTime=T
  Integer Delay1 : Delay  InputProcessing=Inherited  SampleTime=T
  Integer Delay2 : Delay  DelayLength=1  InputProcessing=Inherited  SampleTime=T
  Product{,1..3} (4 alike) : Product  OutDataTypeStr=single  RndMeth=Zero
  "Protect NaNs " : Subsystem
  Protect NaNs1 : Subsystem
  Subtract : Sum  Inputs=3  OutDataTypeStr=single
  Subtract1 : Sum  Inputs=2  OutDataTypeStr=single
  Switch1 : Switch  Criteria=u2 > Threshold  Threshold=0.3  SampleTime=.01
  Int(x) : Outport
  wires:
  Switch1/1 -> Protect NaNs1/1(In1)
  Reset/1 -> Switch1/2
  Constant5/1 -> Switch1/1
  Product3/1 -> Subtract1/2
  Integer Delay2/1 -> Subtract1/1
  Subtract1/1 -> Switch1/3
  Subtract/1 -> Product3/2
  Constant2/1 -> Product3/1
  Product2/1 -> Subtract/3
  Product1/1 -> Subtract/2
  Product/1 -> Subtract/1
  x/1 -> "Protect NaNs "/1(In1)
  Constant3/1 -> Product2/2
  Integer Delay1/1 -> Product2/1
  Integer Delay/1 -> Product1/1
  Constant1/1 -> Product1/2
  Constant/1 -> Product/2
  Protect NaNs1/1(Out1) -> Integer Delay2/1, Int(x)/1
  "Protect NaNs "/1(Out1) -> Integer Delay1/1, Integer Delay/1, Product/1
